simulink model "test_ffts"  (Simulink 6.2)
settings: Solver=ode45  StartTime=0.0  StopTime=300  RelTol=1e-3
undefined symbols (not defined in the file or in its folder): now
libraries: xbsIndex_r3 x1135, fft_library x1, simulink x1
(part 2 of 15)

== system test_ffts/r2_dit_fft ==
  a_in : Inport  Port=1  LatchInput=off
  b_in : Inport  Port=2  LatchInput=off
  sync_in : Inport  Port=3  LatchInput=off
  biplex_bitrev : Subsystem  mask(Biplex Bit Reverse Reorder){log2_size=5, n_bits=14}
      mask prompts: log2_size "Log2 Block Size"; n_bits "Number of Bits"
      mask help: Reorders the input sequence from normal order to bit reverse order (or vise versa).
      settings: AttributesFormatString=size = 32
      mask Help:
      | <pre>
      | Description::
      | 
      | Reorders the input sequence from normal order to bit reverse order (or vise versa).
      | 
      | Mask Parameters::
      | 
      | Log 2 Block Size (log2_size): The base-2 logarithm of the length of one complete input block.
      | This MUST be an integer because the current implementation requires that
      | the input block size MUST be a power of 2.  (aka "N")
      | 
      | Number of Bits (n_bits): Specifies the width of the real/imaginary components.
      | Width of each component is assumed equal.
      | </pre>
  biplex_commutator : Subsystem  mask(Biplex Commutator){log2_size=6, n_bits=14, use_bram=on}
      mask prompts: log2_size "Log2 Block Size"; n_bits "Bit Width"; use_bram "Use BRAM"
      mask help: The biplex commutator commutes the first half of the BloBhi input "block" with the last half of the AloAhi input "block". A "block" is 2^log2_size consecutive samples (i.e. always a power of 2). sync_in precedes the first data input sample by one clock cycle. Overall latency from sync_in to sync_out is 2^(log2_size-1)+1.
      settings: AttributesFormatString=|
      | size = 64
      | complex delay
      mask Help:
      | <pre>
      | Description::
      | 
      | The biplex commutator commutes the first half of the BloBhi input "block"  with the last half
      | of the AloAhi input "block".  A "block" is 2^log2_size consecutive samples (i.e. always a
      | power of 2).
      | 
      | sync_in precedes the first data input sample by one clock cycle.
      | sync_out precedes the corresponding output sample by one clock cycle.
      | Overall latency from sync_in to sync_out is 2^(N-1)+1.
      | 
      | Mask Parameters::
      | 
      | Log 2 Block Size (log2_size): The base-2 logarithm of the length of one complete input block.
      | This MUST be an integer because the current implementation requires that
      | the input block size MUST be a power of 2.  (aka "N")
      | 
      | Bit Width (n_bits): Specifies the width of the real/imaginary components.
      | Width of each component is assumed equal.
      | 
      | Use BRAM (use_bram): Check this checkbox to implement the internal delays using BRAM.
      | If unchecked, the internal delays will be implemented using SLR16 elements.
      | </pre>
  r2_dit_stage_1 : Subsystem  mask(Radix-2 DIT FFT Stage){n_stages=6, cur_stage=1, n_bits=8, bin_pt=7, shift=0, commutator_bram=off, twiddle_bram=off, n_bits_w=9, mult_latency=3, add_latency=1}
      mask prompts: n_stages "Total Stages (2^N points)"; cur_stage "Current Stage"; n_bits "Number of Bits In"; bin_pt "Binary Point In"; shift "Shift Bits"; commutator_bram "Use BRAM for Biplex Commutator"; twiddle_bram "Use BRAM For Twiddle Coefficients"; n_bits_w "Twiddle Coefficient Bitwidth"; mult_latency "Multiplier Latency"; add_latency "Adder Latency"
      mask help: A radix-2 decimation-in-time Fast Fourier Transform stage.
      settings: AttributesFormatString=|
      | stage 1 of 6
      | delay slr
      | twiddle dist
      | shift 0
      mask Help:
      | <pre>
      | Description::
      | 
      | A radix-2 decimation-in-time Fast Fourier Transform stage.
      | 
      | This radix-2 decimation-in-time FFT stage is designed to be daisy chained together
      | to form a multi-stage FFT.  The resulting FFT will have (2^n_stages) points.
      | 
      | The two inputs to the chain are independent complex signals (e.g. A and B).
      | 
      | The two outputs of the last stage of the chain are commuted such that the a_out signal is really
      | the "lower" half of A's transform followed by the "lower" half of B's transform and b_out is really
      | the "upper" half of A's transform followed by the "upper" half of B's transform.  Each half is in bit-reversed order.
      | 
      | If it is desired to have the two halves of A's transform follow each other on the same path and
      | the two halves of B's transform follow each other on the same path, then a_out and b_out can
      | be fed through a biplex_commutator with block size 2^n_stages.  This will result in the "lower"
      | half of A (or B) followed by the "upper" half of A (or B), but note that each half of A (or B)
      | will still remain in bit-reversed order (i.e. each output is bit-reversed in halves; it is not bit reversed
      | in its entirety).
      | 
      | The number of bits for each real and imaginary component grows by one through this stage.
      | If the input bit width is 17 or less, three embedded multipliers will be used per complex multiply.
      | If the input bit width is 18, four embedded multipliers will be used per complex multiply.
      | If the input bit width exceeds 18, then substantially more embedded multipliers will be used
      | per complex multiply.  Enabling "shifting" in some (or all) stages can limit the bit growth
      | to prevent this.
      | 
      | Mask Parameters::
      | 
      | Total Stages (n_stages):  The number of total stages in the FFT.
      | The FFT will have 2^n_stages points.
      | 
      | Current Stage (cur_stage):  The number of the current stage.  Note that stages are counted
      | from 1 to n_stages for DIT (i.e. cur_stage==1 for the first stage).
      | 
      | Number of Bits In (n_bits): Specifies the width of the real/imaginary components of ports
      | a_in and b_in.  Assumed equal for both components.  The real/imaginary components of
      | oorts a_out and b_out will be one bit wider.
      | 
      | Binary Point In (bin_pt): Specifies the binary point position of the real/imaginary
      | components of ports a_in and b_in.  Assumed equal for both components.
      | 
      | Shift Bits (shift): Specifies how many bits to shift (down) by.  A positive value causes
      | the specified number of least significant bits to be dropped.  Usually zero or positive values
      | are used to permit or limit bit growth, but negative values can be used to induce bit growth.
      | 
      | Use BRAM for Biplex Commutator (commutator_bram): Check this checkbox to implement
      | the biplex commutator using BRAM.  If unchecked, the biplex commutator will be implemented
      | using SLR16 elements (i.e. slices).
      | 
      | Use BRAM for Twiddle Coefficients (twiddle_bram): Check this checkbox to store twiddle
      | coefficients in BRAM.  If unchecked, the twiddle coefficients will be sored in distributed
      | memory (i.e. slices).
      | 
      | Twiddle Coefficient Bitwidth (n_bits_w): Specifies the width of the real/imaginary
      | components of the twiddle coefficients.  Assumed equal for both components.
      | 
      | Multiplier Latency (mult_latency): Latency to use for the underlying real multipliers.
      | 
      | Adder Latency (add_latency): Latency to use for the underlying real adders.
      | </pre>
  r2_dit_stage_2 : Subsystem  mask(Radix-2 DIT FFT Stage){n_stages=6, cur_stage=2, n_bits=9, bin_pt=7, shift=0, commutator_bram=off, twiddle_bram=off, n_bits_w=9, mult_latency=3, add_latency=1}
      mask prompts: n_stages "Total Stages (2^N points)"; cur_stage "Current Stage"; n_bits "Number of Bits In"; bin_pt "Binary Point In"; shift "Shift Bits"; commutator_bram "Use BRAM for Biplex Commutator"; twiddle_bram "Use BRAM For Twiddle Coefficients"; n_bits_w "Twiddle Coefficient Bitwidth"; mult_latency "Multiplier Latency"; add_latency "Adder Latency"
      mask help: A radix-2 decimation-in-time Fast Fourier Transform stage.
      settings: AttributesFormatString=|
      | stage 2 of 6
      | delay slr
      | twiddle dist
      | shift 0
      mask Help:
      | <pre>
      | Description::
      | 
      | A radix-2 decimation-in-time Fast Fourier Transform stage.
      | 
      | This radix-2 decimation-in-time FFT stage is designed to be daisy chained together
      | to form a multi-stage FFT.  The resulting FFT will have (2^n_stages) points.
      | 
      | The two inputs to the chain are independent complex signals (e.g. A and B).
      | 
      | The two outputs of the last stage of the chain are commuted such that the a_out signal is really
      | the "lower" half of A's transform followed by the "lower" half of B's transform and b_out is really
      | the "upper" half of A's transform followed by the "upper" half of B's transform.  Each half is in bit-reversed order.
      | 
      | If it is desired to have the two halves of A's transform follow each other on the same path and
      | the two halves of B's transform follow each other on the same path, then a_out and b_out can
      | be fed through a biplex_commutator with block size 2^n_stages.  This will result in the "lower"
      | half of A (or B) followed by the "upper" half of A (or B), but note that each half of A (or B)
      | will still remain in bit-reversed order (i.e. each output is bit-reversed in halves; it is not bit reversed
      | in its entirety).
      | 
      | The number of bits for each real and imaginary component grows by one through this stage.
      | If the input bit width is 17 or less, three embedded multipliers will be used per complex multiply.
      | If the input bit width is 18, four embedded multipliers will be used per complex multiply.
      | If the input bit width exceeds 18, then substantially more embedded multipliers will be used
      | per complex multiply.  Enabling "shifting" in some (or all) stages can limit the bit growth
      | to prevent this.
      | 
      | Mask Parameters::
      | 
      | Total Stages (n_stages):  The number of total stages in the FFT.
      | The FFT will have 2^n_stages points.
      | 
      | Current Stage (cur_stage):  The number of the current stage.  Note that stages are counted
      | from 1 to n_stages for DIT (i.e. cur_stage==1 for the first stage).
      | 
      | Number of Bits In (n_bits): Specifies the width of the real/imaginary components of ports
      | a_in and b_in.  Assumed equal for both components.  The real/imaginary components of
      | oorts a_out and b_out will be one bit wider.
      | 
      | Binary Point In (bin_pt): Specifies the binary point position of the real/imaginary
      | components of ports a_in and b_in.  Assumed equal for both components.
      | 
      | Shift Bits (shift): Specifies how many bits to shift (down) by.  A positive value causes
      | the specified number of least significant bits to be dropped.  Usually zero or positive values
      | are used to permit or limit bit growth, but negative values can be used to induce bit growth.
      | 
      | Use BRAM for Biplex Commutator (commutator_bram): Check this checkbox to implement
      | the biplex commutator using BRAM.  If unchecked, the biplex commutator will be implemented
      | using SLR16 elements (i.e. slices).
      | 
      | Use BRAM for Twiddle Coefficients (twiddle_bram): Check this checkbox to store twiddle
      | coefficients in BRAM.  If unchecked, the twiddle coefficients will be sored in distributed
      | memory (i.e. slices).
      | 
      | Twiddle Coefficient Bitwidth (n_bits_w): Specifies the width of the real/imaginary
      | components of the twiddle coefficients.  Assumed equal for both components.
      | 
      | Multiplier Latency (mult_latency): Latency to use for the underlying real multipliers.
      | 
      | Adder Latency (add_latency): Latency to use for the underlying real adders.
      | </pre>
  r2_dit_stage_3 : Subsystem  mask(Radix-2 DIT FFT Stage){n_stages=6, cur_stage=3, n_bits=10, bin_pt=7, shift=0, commutator_bram=off, twiddle_bram=off, n_bits_w=9, mult_latency=3, add_latency=1}
      mask prompts: n_stages "Total Stages (2^N points)"; cur_stage "Current Stage"; n_bits "Number of Bits In"; bin_pt "Binary Point In"; shift "Shift Bits"; commutator_bram "Use BRAM for Biplex Commutator"; twiddle_bram "Use BRAM For Twiddle Coefficients"; n_bits_w "Twiddle Coefficient Bitwidth"; mult_latency "Multiplier Latency"; add_latency "Adder Latency"
      mask help: A radix-2 decimation-in-time Fast Fourier Transform stage.
      settings: AttributesFormatString=|
      | stage 3 of 6
      | delay slr
      | twiddle dist
      | shift 0
      mask Help:
      | <pre>
      | Description::
      | 
      | A radix-2 decimation-in-time Fast Fourier Transform stage.
      | 
      | This radix-2 decimation-in-time FFT stage is designed to be daisy chained together
      | to form a multi-stage FFT.  The resulting FFT will have (2^n_stages) points.
      | 
      | The two inputs to the chain are independent complex signals (e.g. A and B).
      | 
      | The two outputs of the last stage of the chain are commuted such that the a_out signal is really
      | the "lower" half of A's transform followed by the "lower" half of B's transform and b_out is really
      | the "upper" half of A's transform followed by the "upper" half of B's transform.  Each half is in bit-reversed order.
      | 
      | If it is desired to have the two halves of A's transform follow each other on the same path and
      | the two halves of B's transform follow each other on the same path, then a_out and b_out can
      | be fed through a biplex_commutator with block size 2^n_stages.  This will result in the "lower"
      | half of A (or B) followed by the "upper" half of A (or B), but note that each half of A (or B)
      | will still remain in bit-reversed order (i.e. each output is bit-reversed in halves; it is not bit reversed
      | in its entirety).
      | 
      | The number of bits for each real and imaginary component grows by one through this stage.
      | If the input bit width is 17 or less, three embedded multipliers will be used per complex multiply.
      | If the input bit width is 18, four embedded multipliers will be used per complex multiply.
      | If the input bit width exceeds 18, then substantially more embedded multipliers will be used
      | per complex multiply.  Enabling "shifting" in some (or all) stages can limit the bit growth
      | to prevent this.
      | 
      | Mask Parameters::
      | 
      | Total Stages (n_stages):  The number of total stages in the FFT.
      | The FFT will have 2^n_stages points.
      | 
      | Current Stage (cur_stage):  The number of the current stage.  Note that stages are counted
      | from 1 to n_stages for DIT (i.e. cur_stage==1 for the first stage).
      | 
      | Number of Bits In (n_bits): Specifies the width of the real/imaginary components of ports
      | a_in and b_in.  Assumed equal for both components.  The real/imaginary components of
      | oorts a_out and b_out will be one bit wider.
      | 
      | Binary Point In (bin_pt): Specifies the binary point position of the real/imaginary
      | components of ports a_in and b_in.  Assumed equal for both components.
      | 
      | Shift Bits (shift): Specifies how many bits to shift (down) by.  A positive value causes
      | the specified number of least significant bits to be dropped.  Usually zero or positive values
      | are used to permit or limit bit growth, but negative values can be used to induce bit growth.
      | 
      | Use BRAM for Biplex Commutator (commutator_bram): Check this checkbox to implement
      | the biplex commutator using BRAM.  If unchecked, the biplex commutator will be implemented
      | using SLR16 elements (i.e. slices).
      | 
      | Use BRAM for Twiddle Coefficients (twiddle_bram): Check this checkbox to store twiddle
      | coefficients in BRAM.  If unchecked, the twiddle coefficients will be sored in distributed
      | memory (i.e. slices).
      | 
      | Twiddle Coefficient Bitwidth (n_bits_w): Specifies the width of the real/imaginary
      | components of the twiddle coefficients.  Assumed equal for both components.
      | 
      | Multiplier Latency (mult_latency): Latency to use for the underlying real multipliers.
      | 
      | Adder Latency (add_latency): Latency to use for the underlying real adders.
      | </pre>
  r2_dit_stage_4 : Subsystem  mask(Radix-2 DIT FFT Stage){n_stages=6, cur_stage=4, n_bits=11, bin_pt=7, shift=0, commutator_bram=off, twiddle_bram=off, n_bits_w=9, mult_latency=3, add_latency=1}
      mask prompts: n_stages "Total Stages (2^N points)"; cur_stage "Current Stage"; n_bits "Number of Bits In"; bin_pt "Binary Point In"; shift "Shift Bits"; commutator_bram "Use BRAM for Biplex Commutator"; twiddle_bram "Use BRAM For Twiddle Coefficients"; n_bits_w "Twiddle Coefficient Bitwidth"; mult_latency "Multiplier Latency"; add_latency "Adder Latency"
      mask help: A radix-2 decimation-in-time Fast Fourier Transform stage.
      settings: AttributesFormatString=|
      | stage 4 of 6
      | delay slr
      | twiddle dist
      | shift 0
      mask Help:
      | <pre>
      | Description::
      | 
      | A radix-2 decimation-in-time Fast Fourier Transform stage.
      | 
      | This radix-2 decimation-in-time FFT stage is designed to be daisy chained together
      | to form a multi-stage FFT.  The resulting FFT will have (2^n_stages) points.
      | 
      | The two inputs to the chain are independent complex signals (e.g. A and B).
      | 
      | The two outputs of the last stage of the chain are commuted such that the a_out signal is really
      | the "lower" half of A's transform followed by the "lower" half of B's transform and b_out is really
      | the "upper" half of A's transform followed by the "upper" half of B's transform.  Each half is in bit-reversed order.
      | 
      | If it is desired to have the two halves of A's transform follow each other on the same path and
      | the two halves of B's transform follow each other on the same path, then a_out and b_out can
      | be fed through a biplex_commutator with block size 2^n_stages.  This will result in the "lower"
      | half of A (or B) followed by the "upper" half of A (or B), but note that each half of A (or B)
      | will still remain in bit-reversed order (i.e. each output is bit-reversed in halves; it is not bit reversed
      | in its entirety).
      | 
      | The number of bits for each real and imaginary component grows by one through this stage.
      | If the input bit width is 17 or less, three embedded multipliers will be used per complex multiply.
      | If the input bit width is 18, four embedded multipliers will be used per complex multiply.
      | If the input bit width exceeds 18, then substantially more embedded multipliers will be used
      | per complex multiply.  Enabling "shifting" in some (or all) stages can limit the bit growth
      | to prevent this.
      | 
      | Mask Parameters::
      | 
      | Total Stages (n_stages):  The number of total stages in the FFT.
      | The FFT will have 2^n_stages points.
      | 
      | Current Stage (cur_stage):  The number of the current stage.  Note that stages are counted
      | from 1 to n_stages for DIT (i.e. cur_stage==1 for the first stage).
      | 
      | Number of Bits In (n_bits): Specifies the width of the real/imaginary components of ports
      | a_in and b_in.  Assumed equal for both components.  The real/imaginary components of
      | oorts a_out and b_out will be one bit wider.
      | 
      | Binary Point In (bin_pt): Specifies the binary point position of the real/imaginary
      | components of ports a_in and b_in.  Assumed equal for both components.
      | 
      | Shift Bits (shift): Specifies how many bits to shift (down) by.  A positive value causes
      | the specified number of least significant bits to be dropped.  Usually zero or positive values
      | are used to permit or limit bit growth, but negative values can be used to induce bit growth.
      | 
      | Use BRAM for Biplex Commutator (commutator_bram): Check this checkbox to implement
      | the biplex commutator using BRAM.  If unchecked, the biplex commutator will be implemented
      | using SLR16 elements (i.e. slices).
      | 
      | Use BRAM for Twiddle Coefficients (twiddle_bram): Check this checkbox to store twiddle
      | coefficients in BRAM.  If unchecked, the twiddle coefficients will be sored in distributed
      | memory (i.e. slices).
      | 
      | Twiddle Coefficient Bitwidth (n_bits_w): Specifies the width of the real/imaginary
      | components of the twiddle coefficients.  Assumed equal for both components.
      | 
      | Multiplier Latency (mult_latency): Latency to use for the underlying real multipliers.
      | 
      | Adder Latency (add_latency): Latency to use for the underlying real adders.
      | </pre>
  r2_dit_stage_5 : Subsystem  mask(Radix-2 DIT FFT Stage){n_stages=6, cur_stage=5, n_bits=12, bin_pt=7, shift=0, commutator_bram=off, twiddle_bram=off, n_bits_w=9, mult_latency=3, add_latency=1}
      mask prompts: n_stages "Total Stages (2^N points)"; cur_stage "Current Stage"; n_bits "Number of Bits In"; bin_pt "Binary Point In"; shift "Shift Bits"; commutator_bram "Use BRAM for Biplex Commutator"; twiddle_bram "Use BRAM For Twiddle Coefficients"; n_bits_w "Twiddle Coefficient Bitwidth"; mult_latency "Multiplier Latency"; add_latency "Adder Latency"
      mask help: A radix-2 decimation-in-time Fast Fourier Transform stage.
      settings: AttributesFormatString=|
      | stage 5 of 6
      | delay slr
      | twiddle dist
      | shift 0
      mask Help:
      | <pre>
      | Description::
      | 
      | A radix-2 decimation-in-time Fast Fourier Transform stage.
      | 
      | This radix-2 decimation-in-time FFT stage is designed to be daisy chained together
      | to form a multi-stage FFT.  The resulting FFT will have (2^n_stages) points.
      | 
      | The two inputs to the chain are independent complex signals (e.g. A and B).
      | 
      | The two outputs of the last stage of the chain are commuted such that the a_out signal is really
      | the "lower" half of A's transform followed by the "lower" half of B's transform and b_out is really
      | the "upper" half of A's transform followed by the "upper" half of B's transform.  Each half is in bit-reversed order.
      | 
      | If it is desired to have the two halves of A's transform follow each other on the same path and
      | the two halves of B's transform follow each other on the same path, then a_out and b_out can
      | be fed through a biplex_commutator with block size 2^n_stages.  This will result in the "lower"
      | half of A (or B) followed by the "upper" half of A (or B), but note that each half of A (or B)
      | will still remain in bit-reversed order (i.e. each output is bit-reversed in halves; it is not bit reversed
      | in its entirety).
      | 
      | The number of bits for each real and imaginary component grows by one through this stage.
      | If the input bit width is 17 or less, three embedded multipliers will be used per complex multiply.
      | If the input bit width is 18, four embedded multipliers will be used per complex multiply.
      | If the input bit width exceeds 18, then substantially more embedded multipliers will be used
      | per complex multiply.  Enabling "shifting" in some (or all) stages can limit the bit growth
      | to prevent this.
      | 
      | Mask Parameters::
      | 
      | Total Stages (n_stages):  The number of total stages in the FFT.
      | The FFT will have 2^n_stages points.
      | 
      | Current Stage (cur_stage):  The number of the current stage.  Note that stages are counted
      | from 1 to n_stages for DIT (i.e. cur_stage==1 for the first stage).
      | 
      | Number of Bits In (n_bits): Specifies the width of the real/imaginary components of ports
      | a_in and b_in.  Assumed equal for both components.  The real/imaginary components of
      | oorts a_out and b_out will be one bit wider.
      | 
      | Binary Point In (bin_pt): Specifies the binary point position of the real/imaginary
      | components of ports a_in and b_in.  Assumed equal for both components.
      | 
      | Shift Bits (shift): Specifies how many bits to shift (down) by.  A positive value causes
      | the specified number of least significant bits to be dropped.  Usually zero or positive values
      | are used to permit or limit bit growth, but negative values can be used to induce bit growth.
      | 
      | Use BRAM for Biplex Commutator (commutator_bram): Check this checkbox to implement
      | the biplex commutator using BRAM.  If unchecked, the biplex commutator will be implemented
      | using SLR16 elements (i.e. slices).
      | 
      | Use BRAM for Twiddle Coefficients (twiddle_bram): Check this checkbox to store twiddle
      | coefficients in BRAM.  If unchecked, the twiddle coefficients will be sored in distributed
      | memory (i.e. slices).
      | 
      | Twiddle Coefficient Bitwidth (n_bits_w): Specifies the width of the real/imaginary
      | components of the twiddle coefficients.  Assumed equal for both components.
      | 
      | Multiplier Latency (mult_latency): Latency to use for the underlying real multipliers.
      | 
      | Adder Latency (add_latency): Latency to use for the underlying real adders.
      | </pre>
  r2_dit_stage_6 : Subsystem  mask(Radix-2 DIT FFT Stage){n_stages=6, cur_stage=6, n_bits=13, bin_pt=7, shift=0, commutator_bram=off, twiddle_bram=off, n_bits_w=9, mult_latency=3, add_latency=1}
      mask prompts: n_stages "Total Stages (2^N points)"; cur_stage "Current Stage"; n_bits "Number of Bits In"; bin_pt "Binary Point In"; shift "Shift Bits"; commutator_bram "Use BRAM for Biplex Commutator"; twiddle_bram "Use BRAM For Twiddle Coefficients"; n_bits_w "Twiddle Coefficient Bitwidth"; mult_latency "Multiplier Latency"; add_latency "Adder Latency"
      mask help: A radix-2 decimation-in-time Fast Fourier Transform stage.
      settings: AttributesFormatString=|
      | stage 6 of 6
      | delay slr
      | twiddle dist
      | shift 0
      mask Help:
      | <pre>
      | Description::
      | 
      | A radix-2 decimation-in-time Fast Fourier Transform stage.
      | 
      | This radix-2 decimation-in-time FFT stage is designed to be daisy chained together
      | to form a multi-stage FFT.  The resulting FFT will have (2^n_stages) points.
      | 
      | The two inputs to the chain are independent complex signals (e.g. A and B).
      | 
      | The two outputs of the last stage of the chain are commuted such that the a_out signal is really
      | the "lower" half of A's transform followed by the "lower" half of B's transform and b_out is really
      | the "upper" half of A's transform followed by the "upper" half of B's transform.  Each half is in bit-reversed order.
      | 
      | If it is desired to have the two halves of A's transform follow each other on the same path and
      | the two halves of B's transform follow each other on the same path, then a_out and b_out can
      | be fed through a biplex_commutator with block size 2^n_stages.  This will result in the "lower"
      | half of A (or B) followed by the "upper" half of A (or B), but note that each half of A (or B)
      | will still remain in bit-reversed order (i.e. each output is bit-reversed in halves; it is not bit reversed
      | in its entirety).
      | 
      | The number of bits for each real and imaginary component grows by one through this stage.
      | If the input bit width is 17 or less, three embedded multipliers will be used per complex multiply.
      | If the input bit width is 18, four embedded multipliers will be used per complex multiply.
      | If the input bit width exceeds 18, then substantially more embedded multipliers will be used
      | per complex multiply.  Enabling "shifting" in some (or all) stages can limit the bit growth
      | to prevent this.
      | 
      | Mask Parameters::
      | 
      | Total Stages (n_stages):  The number of total stages in the FFT.
      | The FFT will have 2^n_stages points.
      | 
      | Current Stage (cur_stage):  The number of the current stage.  Note that stages are counted
      | from 1 to n_stages for DIT (i.e. cur_stage==1 for the first stage).
      | 
      | Number of Bits In (n_bits): Specifies the width of the real/imaginary components of ports
      | a_in and b_in.  Assumed equal for both components.  The real/imaginary components of
      | oorts a_out and b_out will be one bit wider.
      | 
      | Binary Point In (bin_pt): Specifies the binary point position of the real/imaginary
      | components of ports a_in and b_in.  Assumed equal for both components.
      | 
      | Shift Bits (shift): Specifies how many bits to shift (down) by.  A positive value causes
      | the specified number of least significant bits to be dropped.  Usually zero or positive values
      | are used to permit or limit bit growth, but negative values can be used to induce bit growth.
      | 
      | Use BRAM for Biplex Commutator (commutator_bram): Check this checkbox to implement
      | the biplex commutator using BRAM.  If unchecked, the biplex commutator will be implemented
      | using SLR16 elements (i.e. slices).
      | 
      | Use BRAM for Twiddle Coefficients (twiddle_bram): Check this checkbox to store twiddle
      | coefficients in BRAM.  If unchecked, the twiddle coefficients will be sored in distributed
      | memory (i.e. slices).
      | 
      | Twiddle Coefficient Bitwidth (n_bits_w): Specifies the width of the real/imaginary
      | components of the twiddle coefficients.  Assumed equal for both components.
      | 
      | Multiplier Latency (mult_latency): Latency to use for the underlying real multipliers.
      | 
      | Adder Latency (add_latency): Latency to use for the underlying real adders.
      | </pre>
  a_out : Outport
  b_out : Outport  Port=2
  sync_out : Outport  Port=3
  wires:
  a_in/1 -> r2_dit_stage_1/1(a_in)
  b_in/1 -> r2_dit_stage_1/2(b_in)
  sync_in/1 -> r2_dit_stage_1/3(sync_in)
  r2_dit_stage_1/1(a_out) -> r2_dit_stage_2/1(a_in)
  r2_dit_stage_1/2(b_out) -> r2_dit_stage_2/2(b_in)
  r2_dit_stage_1/3(sync_out) -> r2_dit_stage_2/3(sync_in)
  r2_dit_stage_2/1(a_out) -> r2_dit_stage_3/1(a_in)
  r2_dit_stage_2/2(b_out) -> r2_dit_stage_3/2(b_in)
  r2_dit_stage_2/3(sync_out) -> r2_dit_stage_3/3(sync_in)
  r2_dit_stage_3/1(a_out) -> r2_dit_stage_4/1(a_in)
  r2_dit_stage_3/2(b_out) -> r2_dit_stage_4/2(b_in)
  r2_dit_stage_3/3(sync_out) -> r2_dit_stage_4/3(sync_in)
  r2_dit_stage_4/1(a_out) -> r2_dit_stage_5/1(a_in)
  r2_dit_stage_4/2(b_out) -> r2_dit_stage_5/2(b_in)
  r2_dit_stage_4/3(sync_out) -> r2_dit_stage_5/3(sync_in)
  r2_dit_stage_5/1(a_out) -> r2_dit_stage_6/1(a_in)
  r2_dit_stage_5/2(b_out) -> r2_dit_stage_6/2(b_in)
  r2_dit_stage_5/3(sync_out) -> r2_dit_stage_6/3(sync_in)
  r2_dit_stage_6/1(a_out) -> biplex_commutator/1(AloAhi)
  r2_dit_stage_6/2(b_out) -> biplex_commutator/2(BloBhi)
  r2_dit_stage_6/3(sync_out) -> biplex_commutator/3(sync_in)
  biplex_commutator/1(AloBlo) -> biplex_bitrev/1(a_in)
  biplex_commutator/2(AhiBhi) -> biplex_bitrev/2(b_in)
  biplex_commutator/3(sync_out) -> biplex_bitrev/3(sync_in)
  biplex_bitrev/1(a_out) -> a_out/1
  biplex_bitrev/2(b_out) -> b_out/1
  biplex_bitrev/3(sync_out) -> sync_out/1
